simulink model "sg_IK"  (R2021b)
settings: Solver=ode4  StartTime=0.0  StopTime=10  FixedStep=Ts  RelTol=1e-3  EnableMultiTasking=on
model workspace (MAT data in the model file):
  BList = [0  0  0  0  0; 0  1  -1  1  0; -1  0  0  0  1; 0  1.41  -0.25  0  0; -2.61918  0  0  0  0; 0  -2.26918  2.26918  0  0]
  M = [1  0  0  2.61918; 0  1  0  0; 0  0  1  2.24; 0  0  0  1]
  Manual_State_Switch = 0
  Operation_Mode = 2
  SList = [0  0  0  0  0; 0  1  -1  1  0; -1  0  0  0  1; 0  -0.83  1.99  -2.24  0; 0  0  0  0  -2.61918; 0  0.35  -0.35  2.61918  0]
  State_Mode_Selector = 2
  Traj_method = 1
  Winch_EnableHeaveComp = 0
  Winch_NewCmd = 0
  Winch_PosRef = 10
  controlMode = 2
  new_command_traj = 0
  v_max = 0
  x_coordinate_traj = 0
  y_coordinate_traj = 0
  z_coordinate_traj = 0
values from neighbouring files (symbols this model uses):
  Ts = 1e-3    (= 0.001)    [sg_IK_build.m]    (also in sg_IK_startup.m)
libraries: slpidlib x5, slrealtimeutilitieslib x3, slrealtimeiplib x3, dspfdesign x1, simulink x1
(part 1 of 2)
settings Model: SimulationMode=external  Creator=ronnyl10  LastModifiedBy=Thoma
settings SolverCC: ConcurrentTasks=on  AlgebraicLoopSolver=TrustRegion  PositivePriorityOrder=on  AutoInsertRateTranBlk=on  InsertRTBMode=Never (minimum delay)
settings DataIOCC: ExternalInput=ds  SaveFormat=Array  SaveState=on  InspectSignalLogs=on  SignalLoggingName=logsOut
settings OptimizationCC: BlockReduction=off  BooleanDataType=off  OptimizeBlockIOStorage=off  BufferReuse=off  GlobalBufferReuse=off  ExpressionFolding=off  LocalBlockOutputs=off  InitFltsAndDblsToZero=on  OptimizeDataStoreBuffers=off  BusAssignmentInplaceUpdate=off
settings DebuggingCC: SaveWithParameterizedLinksMsg=none  UnderspecifiedInitializationDetection=Classic  MergeDetectMultiDrivingBlocksExec=none  CheckExecutionContextPreStartOutputMsg=on  SignalResolutionControl=TryResolveAllWithWarning  TasksWithSamePriorityMsg=none  SFUnexpectedBacktrackingDiag=warning  SFNoUnconditionalDefaultTransitionDiag=warning  SFExecutionAtInitializationDiag=none  SFMachineParentedDataDiag=warning  ArithmeticOperatorsInVariantConditions=warning
settings HardwareCC: ProdBitPerLong=64  ProdLongLongMode=on  ProdHWDeviceType=Intel->x86-64 (Linux 64)
settings ModelReferenceCC: PropagateSignalLabelsOutOfModel=off
settings SFSimCC: SimUseLocalCustomCode=off  SimTargetLang=C++
settings RTWCC: Description=Simulink Real-Time  SystemTargetFile=slrealtime.tlc  TemplateMakefile=slrealtime_default_tmf  RTWVerbose=off  RTWUseLocalCustomCode=off  Toolchain=Simulink Real-Time Toolchain  BuildConfiguration=Faster Runs  CodeExecutionProfiling=on  TargetLang=C++
settings CodeAppCC: StateflowObjectComments=on
settings SimulinkRealTimeTargetCC: MATLABClassNameForMDSCustomization=Simulink.SoftwareTarget.GRTCustomization  UseGCCFastMath=on
settings ConfigComp: CovEnable=on  RecordCoverage=on  CovMetricSettings=dw  CovSaveCumulativeToWorkspaceVar=on  CovSaveSingleToWorkspaceVar=on  CovModelRefEnable=on  CovExternalEMLEnable=off  CovSFcnEnable=off  PLC_TargetIDE=codesys23  PLC_MultiTBSigbuilderTimeRange=off  PLC_InlineEnumCastFunction=off
settings SimscapeCC: SimscapeLogType=local

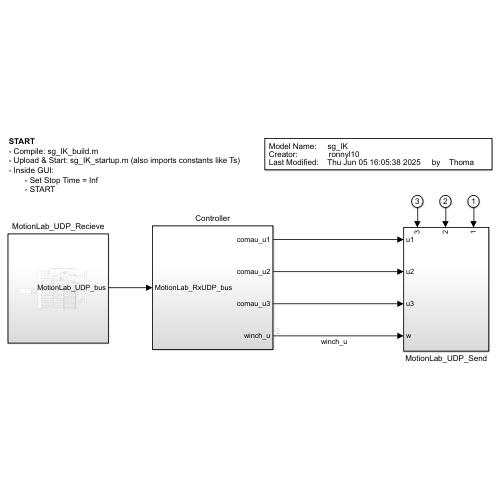
[thumbnail: Simulink's stored preview of the top-level diagram]
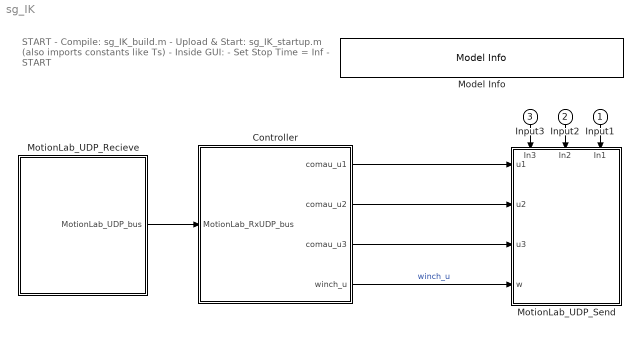
== system sg_IK ==
  note: START
      | - Compile: sg_IK_build.m
      | - Upload & Start: sg_IK_startup.m (also imports constants like Ts)
      | - Inside GUI:
      | - Set Stop Time = Inf
      | - START
  Input1 : Inport  OutDataTypeStr=uint32
  Input2 : Inport  Port=2  OutDataTypeStr=single
  Input3 : Inport  Port=3  OutDataTypeStr=single
  Controller : Subsystem
  Model Info : simulink/Model-Wide Utilities/Model Info  Frame=on  DisplayStringWithTags=|  HorizontalTextAlignment=Left  LeftAlignmentValue=0.02
      | Model Name:     %<ModelName>
      | Creator:              %<Creator>
      | Last Modified:    %<LastModificationDate>     by    %<LastModifiedBy>
  MotionLab_UDP_Recieve : Subsystem
      settings: PortSchema="{\"entries\":[{\"content\":{\"sides\":[{\"content\":{\"connectorIds\":[\"Out1\"]},\"type\":\"ConnectorPlacement.EquallySpacedRectSide\",\"uuid\":\"c59011e9-d1b7-40a2-9e4f-4209006e1514\"},{\"content\":{\"connectorIds\":[],\"side\":\"RIGHT\"},\"type\":\"ConnectorPlacement.EquallySpacedRectSide\",\"uuid\":\"30246177-6108-4738-a92b-25ec176522a5\"},{\"content\":{\"connectorIds\":[],\"side\":\"TOP\"},\"type\":\"ConnectorPlacement.EquallySpacedRectSide\",\"uuid\":\"73bbeb10-9b84-43ee-922e-4b95a3463826\"}]},\"type\":\"ConnectorPlacement.EquallySpacedConnector\",\"uuid\":\"322088d5-facc-406b-b4f7-14c8360d1d37\"}],\"packageUris\":[\"http://schema.mathworks.com/mf0/Connector/R2020b\"],\"version\":\"1.0\"}"
  MotionLab_UDP_Send : Subsystem
      settings: PortSchema="{\"entries\":[{\"content\":{\"sides\":[{\"content\":{\"connectorIds\":[\"In1\",\"In2\",\"In3\"]},\"type\":\"ConnectorPlacement.EquallySpacedRectSide\",\"uuid\":\"2ce4a3a0-ffcc-43d7-9a0a-8eda699e79f7\"},{\"content\":{\"connectorIds\":[],\"side\":\"RIGHT\"},\"type\":\"ConnectorPlacement.EquallySpacedRectSide\",\"uuid\":\"6b0835cb-1c02-4104-b44f-3bd25ad1f1a4\"},{\"content\":{\"connectorIds\":[],\"side\":\"TOP\"},\"type\":\"ConnectorPlacement.EquallySpacedRectSide\",\"uuid\":\"5708f016-a603-4602-bfb0-c60eac1ca3fe\"},{\"content\":{\"connectorIds\":[\"In4\",\"In5\",\"In6\",\"In7\"],\"side\":\"BOTTOM\"},\"type\":\"ConnectorPlacement.EquallySpacedRectSide\",\"uuid\":\"ec76ed57-869b-40d0-9db7-9ec796597bae\"}]},\"type\":\"ConnectorPlacement.EquallySpacedConnector\",\"uuid\":\"dfe3046e-e9d4-4a64-bd13-28ebfaf09d3c\"}],\"packageUris\":[\"http://schema.mathworks.com/mf0/Connector/R2020b\"],\"version\":\"1.0\"}"
  wires:
  Input1/1 -> MotionLab_UDP_Send/1(In1)
  Input3/1 -> MotionLab_UDP_Send/3(In3)
  Input2/1 -> MotionLab_UDP_Send/2(In2)
  Controller/3(comau_u3) -> MotionLab_UDP_Send/6(u3)
  Controller/2(comau_u2) -> MotionLab_UDP_Send/5(u2)
  Controller/1(comau_u1) -> MotionLab_UDP_Send/4(u1)
  Controller/4(winch_u) -> MotionLab_UDP_Send/7(w)  "winch_u"
  MotionLab_UDP_Recieve/1(MotionLab_UDP_bus) -> Controller/1(MotionLab_RxUDP_bus)

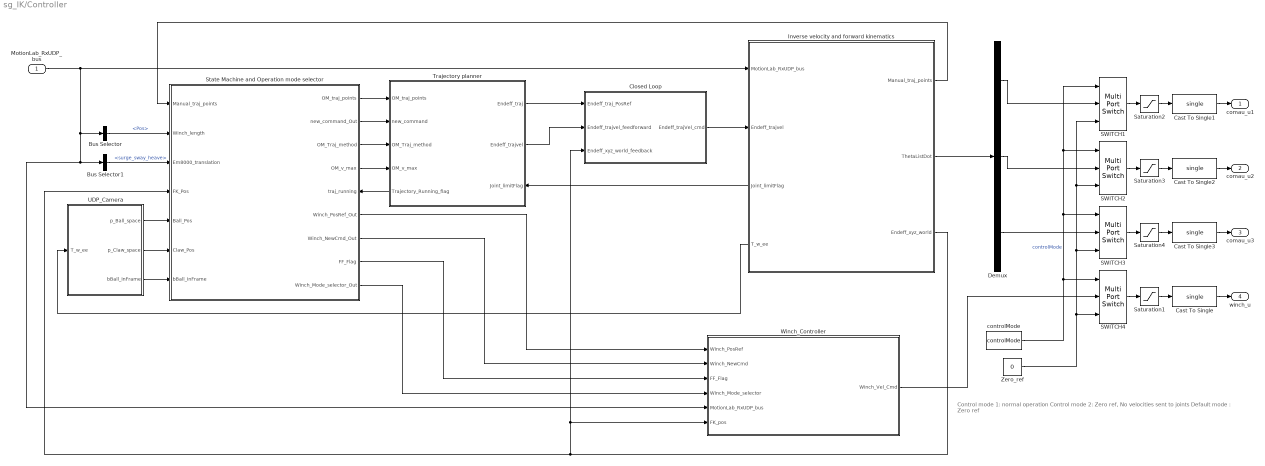
== system sg_IK/Controller ==
  note: Control mode 1: normal operation
      | Control mode 2: Zero ref, No velocities sent to joints
      | Default mode : Zero ref
  MotionLab_RxUDP_bus : Inport
  Bus Selector : BusSelector  OutputSignals=Comau_winch.Pos
  Bus Selector1 : BusSelector  OutputSignals=Em8000.surge_sway_heave
  Cast To Single{,1..3} (4 alike) : DataTypeConversion  OutDataTypeStr=single
  Closed Loop : Subsystem
  Demux : Demux  Outputs=3
  Inverse velocity and forward kinematics : Subsystem
      settings: PortSchema="{\"entries\":[{\"content\":{\"sides\":[{\"content\":{\"connectorIds\":[\"In1\",\"In2\",\"Out4\",\"Out5\"]},\"type\":\"ConnectorPlacement.EquallySpacedRectSide\",\"uuid\":\"551e022a-d0a0-4fc0-a0b4-a546033360d6\"},{\"content\":{\"connectorIds\":[\"Out1\",\"Out2\",\"Out3\"],\"side\":\"RIGHT\"},\"type\":\"ConnectorPlacement.EquallySpacedRectSide\",\"uuid\":\"f9bd0db6-08fd-404e-abaa-5ee6a95abaa6\"},{\"content\":{\"connectorIds\":[],\"side\":\"TOP\"},\"type\":\"ConnectorPlacement.EquallySpacedRectSide\",\"uuid\":\"fe065caa-714c-4067-9577-83ed1adbb3af\"}]},\"type\":\"ConnectorPlacement.EquallySpacedConnector\",\"uuid\":\"f9e419c5-0059-4eec-ae0b-901e5e66b203\"}],\"packageUris\":[\"http://schema.mathworks.com/mf0/Connector/R2020b\"],\"version\":\"1.0\"}"
  SWITCH1 : MultiPortSwitch  Inputs=2
  SWITCH2 : MultiPortSwitch  Inputs=2
  SWITCH3 : MultiPortSwitch  Inputs=2
  SWITCH4 : MultiPortSwitch  Inputs=2  DataPortIndices={1,3}
  Saturation{1..4} (4 alike) : Saturate  UpperLimit=1  LowerLimit=-1
  State Machine and Operation mode selector : Subsystem
      settings: PortSchema="{\"entries\":[{\"content\":{\"sides\":[{\"content\":{\"connectorIds\":[\"In1\",\"In2\",\"In3\",\"In4\",\"In5\",\"In6\",\"In7\"]},\"type\":\"ConnectorPlacement.EquallySpacedRectSide\",\"uuid\":\"2c888d26-e36d-4bcc-8a24-3953247e7d64\"},{\"content\":{\"connectorIds\":[\"Out1\",\"Out2\",\"Out3\",\"Out4\",\"In8\",\"Out5\",\"Out6\",\"Out7\",\"Out8\"],\"side\":\"RIGHT\"},\"type\":\"ConnectorPlacement.EquallySpacedRectSide\",\"uuid\":\"56a7b940-10db-4de5-8f34-3a22dd933015\"},{\"content\":{\"connectorIds\":[],\"side\":\"TOP\"},\"type\":\"ConnectorPlacement.EquallySpacedRectSide\",\"uuid\":\"a958dc8e-1891-4e1e-9098-eeadf2f07291\"}]},\"type\":\"ConnectorPlacement.EquallySpacedConnector\",\"uuid\":\"dcd22044-37ce-4261-aa6a-e53076204f46\"}],\"packageUris\":[\"http://schema.mathworks.com/mf0/Connector/R2020b\"],\"version\":\"1.0\"}"
  Trajectory planner : Subsystem
      settings: PortSchema="{\"entries\":[{\"content\":{\"sides\":[{\"content\":{\"connectorIds\":[\"In1\",\"In2\",\"In3\",\"In4\",\"Out3\"]},\"type\":\"ConnectorPlacement.EquallySpacedRectSide\",\"uuid\":\"e3993239-e7e3-4a56-997d-74b7ac6f065a\"},{\"content\":{\"connectorIds\":[\"Out1\",\"Out2\",\"In5\"],\"side\":\"RIGHT\"},\"type\":\"ConnectorPlacement.EquallySpacedRectSide\",\"uuid\":\"19f001ca-a0d0-47d2-9d98-171e423b1018\"},{\"content\":{\"connectorIds\":[],\"side\":\"TOP\"},\"type\":\"ConnectorPlacement.EquallySpacedRectSide\",\"uuid\":\"ee801cb8-1bce-4750-91c9-73da0ed4f570\"}]},\"type\":\"ConnectorPlacement.EquallySpacedConnector\",\"uuid\":\"affe814f-e012-4d2a-a83d-4eb69c1cbd99\"}],\"packageUris\":[\"http://schema.mathworks.com/mf0/Connector/R2020b\"],\"version\":\"1.0\"}"
  UDP_Camera : Subsystem
  Winch_Controller : Subsystem
  Zero_ref : Constant  Value=0  OutDataTypeStr=double
  controlMode : Constant  Value=controlMode  OutDataTypeStr=double
  comau_u1 : Outport
  comau_u2 : Outport  Port=2
  comau_u3 : Outport  Port=3
  winch_u : Outport  Port=4
  wires:
  Saturation1/1 -> Cast To Single/1
  Zero_ref/1 -> SWITCH1/3, SWITCH2/3, SWITCH3/3, SWITCH4/3
  SWITCH4/1 -> Saturation1/1
  SWITCH1/1 -> Saturation2/1
  SWITCH2/1 -> Saturation3/1
  SWITCH3/1 -> Saturation4/1
  controlMode/1 -> SWITCH1/1, SWITCH2/1, SWITCH3/1, SWITCH4/1  "controlMode"
  Cast To Single/1 -> winch_u/1
  Cast To Single3/1 -> comau_u3/1
  Saturation4/1 -> Cast To Single3/1
  Saturation3/1 -> Cast To Single2/1
  Cast To Single2/1 -> comau_u2/1
  Saturation2/1 -> Cast To Single1/1
  Cast To Single1/1 -> comau_u1/1
  Demux/1 -> SWITCH1/2
  Demux/2 -> SWITCH2/2
  Demux/3 -> SWITCH3/2
  Winch_Controller/1(Winch_Vel_Cmd) -> SWITCH4/2
  Inverse velocity and forward kinematics/3(Endeff_xyz_world) -> Winch_Controller/6(FK_pos), Closed Loop/3(Endeff_xyz_world_feedback), State Machine and Operation mode selector/4(FK_Pos)
  MotionLab_RxUDP_bus/1 -> Winch_Controller/5(MotionLab_RxUDP_bus), Bus Selector1/1, Bus Selector/1, Inverse velocity and forward kinematics/1(MotionLab_RxUDP_bus)
  Inverse velocity and forward kinematics/2(ThetaListDot) -> Demux/1
  Inverse velocity and forward kinematics/4(Joint_limitFlag) -> Trajectory planner/5(Joint_limitFlag)
  Trajectory planner/2(Endeff_trajvel) -> Closed Loop/2(Endeff_trajvel_feedforward)
  Inverse velocity and forward kinematics/1(Manual_traj_points) -> State Machine and Operation mode selector/1(Manual_traj_points)
  Trajectory planner/3(Trajectory_Running_flag) -> State Machine and Operation mode selector/8(traj_running)
  UDP_Camera/1(p_Ball_space) -> State Machine and Operation mode selector/5(Ball_Pos)
  UDP_Camera/2(p_Claw_space) -> State Machine and Operation mode selector/6(Claw_Pos)
  UDP_Camera/3(bBall_InFrame) -> State Machine and Operation mode selector/7(bBall_InFrame)
  State Machine and Operation mode selector/1(OM_traj_points) -> Trajectory planner/1(OM_traj_points)
  State Machine and Operation mode selector/2(new_command_Out) -> Trajectory planner/2(new_command)
  State Machine and Operation mode selector/3(OM_Traj_method) -> Trajectory planner/3(OM_Traj_method)
  State Machine and Operation mode selector/4(OM_v_max) -> Trajectory planner/4(OM_v_max)
  State Machine and Operation mode selector/5(Winch_PosRef_Out) -> Winch_Controller/1(Winch_PosRef)
  State Machine and Operation mode selector/6(Winch_NewCmd_Out) -> Winch_Controller/2(Winch_NewCmd)
  State Machine and Operation mode selector/7(FF_Flag) -> Winch_Controller/3(FF_Flag)
  Bus Selector/1 -> State Machine and Operation mode selector/2(Winch_length)  "<Pos>"
  Inverse velocity and forward kinematics/5(T_w_ee) -> UDP_Camera/1(T_w_ee)
  State Machine and Operation mode selector/8(Winch_Mode_selector_Out) -> Winch_Controller/4(Winch_Mode_selector)
  Bus Selector1/1 -> State Machine and Operation mode selector/3(Em8000_translation)  "<surge_sway_heave>"
  Closed Loop/1(Endeff_trajVel_cmd) -> Inverse velocity and forward kinematics/2(Endeff_trajvel)
  Trajectory planner/1(Endeff_traj) -> Closed Loop/1(Endeff_traj_PosRef)

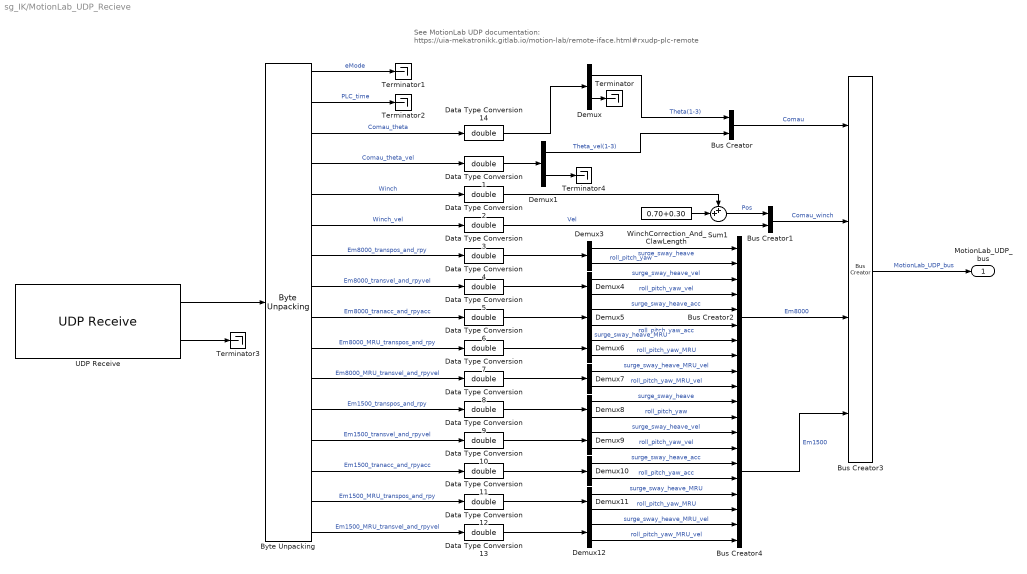
== system sg_IK/MotionLab_UDP_Recieve ==
  note: See MotionLab UDP documentation:
      | https://uia-mekatronikk.gitlab.io/motion-lab/remote-iface.html#rxudp-plc-remote
  Bus Creator : BusCreator  Inputs=2
  Bus Creator1 : BusCreator  Inputs=2
  Bus Creator2 : BusCreator  Inputs=10
  Bus Creator3 : BusCreator  Inputs=4
  Bus Creator4 : BusCreator  Inputs=10
  Byte Unpacking : slrealtimeutilitieslib/Byte Unpacking  MaskUnpackedDataTypes={'uint32', 'single', 'single', 'single', 'single', 'single', 'single', 'single', 'single', 'single', 'single', 'single', 'single', 'single', 'single', 'single'}  MaskUnpackedDataSizes={[1], [1], [6], [6], [1], [1], [6], [6], [6], [6], [6], [6], [6], [6], [6], [6]}  MaskAlignment=1
      settings: SourceProductBaseCode=XP
  Data Type Conversion{1..14} (14 alike) : DataTypeConversion  OutDataTypeStr=double
  Demux{,1,3..12} (12 alike) : Demux  Outputs=2
  Sum1 : Sum  Inputs=++|
  Terminator{,1..4} (5 alike) : Terminator
  UDP Receive : slrealtimeiplib/UDP Receive  useHostTargetConn=on  ipAddress=192.168.90.60  localPort=50060  rcvWidth=304  rcvFmAny=on  fmAddress=192.168.90.50  sampleTime=Ts
      settings: SourceProductBaseCode=XP
  WinchCorrection_And_ClawLength : Constant  Value=0.70+0.30
  MotionLab_UDP_bus : Outport
  wires:
  Byte Unpacking/14 -> Data Type Conversion11/1  "Em1500_tranacc_and_rpyacc"
  Byte Unpacking/11 -> Data Type Conversion8/1  "Em8000_MRU_transvel_and_rpyvel"
  Byte Unpacking/12 -> Data Type Conversion9/1  "Em1500_transpos_and_rpy"
  Byte Unpacking/8 -> Data Type Conversion5/1  "Em8000_transvel_and_rpyvel"
  Demux5/1 -> Bus Creator2/5  "surge_sway_heave_acc"
  Byte Unpacking/2 -> Terminator2/1  "PLC_time"
  Data Type Conversion6/1 -> Demux5/1
  Byte Unpacking/16 -> Data Type Conversion13/1  "Em1500_MRU_transvel_and_rpyvel"
  Byte Unpacking/3 -> Data Type Conversion14/1  "Comau_theta"
  Demux9/1 -> Bus Creator4/3  "surge_sway_heave_vel"
  Data Type Conversion7/1 -> Demux6/1
  Byte Unpacking/4 -> Data Type Conversion1/1  "Comau_theta_vel"
  Data Type Conversion12/1 -> Demux11/1
  Data Type Conversion13/1 -> Demux12/1
  Byte Unpacking/5 -> Data Type Conversion2/1  "Winch"
  Data Type Conversion11/1 -> Demux10/1
  Demux4/1 -> Bus Creator2/3  "surge_sway_heave_vel"
  Byte Unpacking/13 -> Data Type Conversion10/1  "Em1500_transvel_and_rpyvel"
  Byte Unpacking/9 -> Data Type Conversion6/1  "Em8000_tranacc_and_rpyacc"
  Data Type Conversion8/1 -> Demux7/1
  Data Type Conversion5/1 -> Demux4/1
  Demux12/2 -> Bus Creator4/10  "roll_pitch_yaw_MRU_vel"
  Data Type Conversion9/1 -> Demux8/1
  Byte Unpacking/7 -> Data Type Conversion4/1  "Em8000_transpos_and_rpy"
  Bus Creator3/1 -> MotionLab_UDP_bus/1  "MotionLab_UDP_bus"
  Data Type Conversion3/1 -> Bus Creator1/2  "Vel"
  Byte Unpacking/1 -> Terminator1/1  "eMode"
  Demux9/2 -> Bus Creator4/4  "roll_pitch_yaw_vel"
  Demux7/2 -> Bus Creator2/10  "roll_pitch_yaw_MRU_vel"
  Demux8/2 -> Bus Creator4/2  "roll_pitch_yaw"
  Data Type Conversion4/1 -> Demux3/1
  UDP Receive/2 -> Terminator3/1
  Byte Unpacking/10 -> Data Type Conversion7/1  "Em8000_MRU_transpos_and_rpy"
  Bus Creator1/1 -> Bus Creator3/2  "Comau_winch"
  Demux6/2 -> Bus Creator2/8  "roll_pitch_yaw_MRU"
  Demux12/1 -> Bus Creator4/9  "surge_sway_heave_MRU_vel"
  Demux5/2 -> Bus Creator2/6  "roll_pitch_yaw_acc"
  Demux11/2 -> Bus Creator4/8  "roll_pitch_yaw_MRU"
  Byte Unpacking/6 -> Data Type Conversion3/1  "Winch_vel"
  Demux11/1 -> Bus Creator4/7  "surge_sway_heave_MRU"
  Demux10/1 -> Bus Creator4/5  "surge_sway_heave_acc"
  Demux3/1 -> Bus Creator2/1  "surge_sway_heave"
  Demux10/2 -> Bus Creator4/6  "roll_pitch_yaw_acc"
  Demux7/1 -> Bus Creator2/9  "surge_sway_heave_MRU_vel"
  Bus Creator2/1 -> Bus Creator3/3  "Em8000"
  Demux/2 -> Terminator/1
  Sum1/1 -> Bus Creator1/1  "Pos"
  Bus Creator4/1 -> Bus Creator3/4  "Em1500"
  Data Type Conversion10/1 -> Demux9/1
  WinchCorrection_And_ClawLength/1 -> Sum1/2
  Demux4/2 -> Bus Creator2/4  "roll_pitch_yaw_vel"
  Byte Unpacking/15 -> Data Type Conversion12/1  "Em1500_MRU_transpos_and_rpy"
  Demux3/2 -> Bus Creator2/2  "roll_pitch_yaw"
  Demux1/1 -> Bus Creator/2  "Theta_vel(1-3)"
  UDP Receive/1 -> Byte Unpacking/1
  Bus Creator/1 -> Bus Creator3/1  "Comau"
  Demux/1 -> Bus Creator/1  "Theta(1-3)"
  Demux8/1 -> Bus Creator4/1  "surge_sway_heave"
  Data Type Conversion14/1 -> Demux/1
  Demux6/1 -> Bus Creator2/7  "surge_sway_heave_MRU"
  Data Type Conversion2/1 -> Sum1/1
  Demux1/2 -> Terminator4/1
  Data Type Conversion1/1 -> Demux1/1

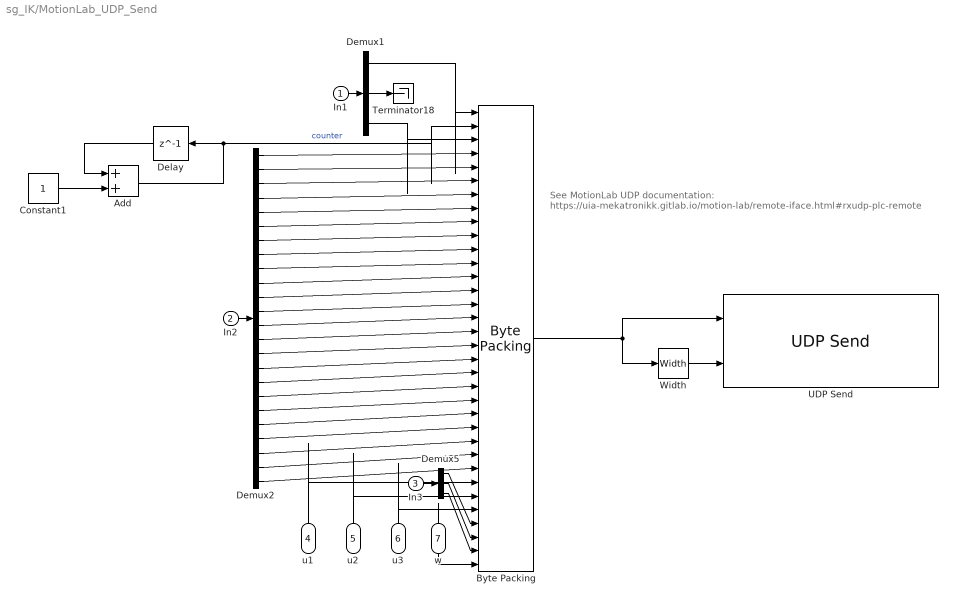
== system sg_IK/MotionLab_UDP_Send ==
  note: See MotionLab UDP documentation:
      | https://uia-mekatronikk.gitlab.io/motion-lab/remote-iface.html#rxudp-plc-remote
  In1 : Inport
  In2 : Inport  Port=2
  In3 : Inport  Port=3
  u1 : Inport  Port=4
  u2 : Inport  Port=5
  u3 : Inport  Port=6
  w : Inport  Port=7
  Add : Sum
  Byte Packing : slrealtimeutilitieslib/Byte Packing  MaskPackedDataType=uint8  MaskUnpackedDataTypes={'uint32', 'uint32', 'uint32', 'single', 'single', 'single', 'single', 'single', 'single', 'single', 'single', 'single', 'single', 'single', 'single', 'single', 'single', 'single', 'single', 'single', 'single', 'single', 'single', 'single', 'single', 'single', 'single', 'single', 'single', 'single', 'single', 'single', 'single', 'single'}  MaskAlignment=1
  Constant1 : Constant  OutDataTypeStr=uint32
  Delay : Delay  DelayLength=1
  Demux1 : Demux  Outputs=3
  Demux2 : Demux  Outputs=24
  Demux5 : Demux  Outputs=3
  Terminator18 : Terminator
  UDP Send : slrealtimeiplib/UDP Send  useHostTargetConn=on  toAddress=192.168.90.50  toPort=50050  sampleTime=Ts  localPort=11000
      settings: SourceProductBaseCode=XP
  Width : Width
  wires:
  Demux2/19 -> Byte Packing/22
  Demux2/21 -> Byte Packing/24
  u3/1 -> Byte Packing/30
  Demux2/2 -> Byte Packing/5
  u2/1 -> Byte Packing/29
  Demux5/1 -> Byte Packing/31
  Demux5/2 -> Byte Packing/32
  Demux1/3 -> Byte Packing/3
  In2/1 -> Demux2/1
  Demux2/22 -> Byte Packing/25
  Demux2/1 -> Byte Packing/4
  Demux2/15 -> Byte Packing/18
  Demux2/18 -> Byte Packing/21
  Delay/1 -> Add/1
  Demux2/24 -> Byte Packing/27
  Demux1/2 -> Terminator18/1
  In1/1 -> Demux1/1
  Demux2/5 -> Byte Packing/8
  Add/1 -> Byte Packing/2, Delay/1  "counter"
  Constant1/1 -> Add/2
  Demux2/6 -> Byte Packing/9
  Demux2/9 -> Byte Packing/12
  Demux2/10 -> Byte Packing/13
  Demux2/20 -> Byte Packing/23
  Demux2/8 -> Byte Packing/11
  Demux2/12 -> Byte Packing/15
  Demux2/23 -> Byte Packing/26
  Demux2/16 -> Byte Packing/19
  Demux1/1 -> Byte Packing/1
  Demux5/3 -> Byte Packing/33
  Demux2/3 -> Byte Packing/6
  Demux2/11 -> Byte Packing/14
  Demux2/7 -> Byte Packing/10
  Demux2/4 -> Byte Packing/7
  Demux2/13 -> Byte Packing/16
  Demux2/17 -> Byte Packing/20
  Demux2/14 -> Byte Packing/17
  u1/1 -> Byte Packing/28
  In3/1 -> Demux5/1
  w/1 -> Byte Packing/34
  Byte Packing/1 -> Width/1, UDP Send/1
  Width/1 -> UDP Send/2

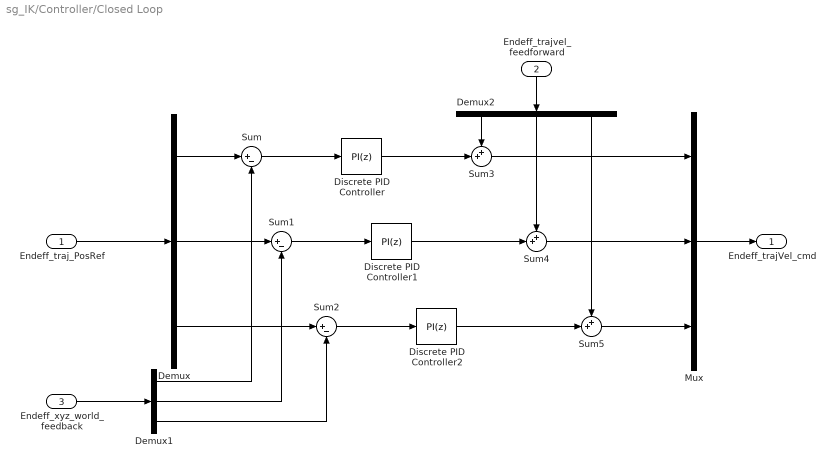
== system sg_IK/Controller/Closed Loop ==
  Endeff_traj_PosRef : Inport
  Endeff_trajvel_feedforward : Inport  Port=2
  Endeff_xyz_world_feedback : Inport  Port=3
  Demux : Demux  Outputs=3
  Demux1 : Demux  Outputs=3
  Demux2 : Demux  Outputs=3
  Discrete PID Controller : slpidlib/PID Controller  Controller=PI  Form=Parallel  TimeDomain=Discrete-time  UseExternalTs=off  SampleTime=Ts  IntegratorMethod=Forward Euler  FilterMethod=Forward Euler  ControllerParametersSource=internal  P=0.25  I=0.0125  D=0  UseFilter=on  N=100  TunerSelectOption=Transfer Function Based (PID Tuner App)  InitialConditionSource=internal  InitialConditionForIntegrator=0  InitialConditionForFilter=0  DifferentiatorICPrevScaledInput=0  ExternalReset=none  TrackingMode=off  Kt=1  LimitOutput=on  SatLimitsSource=internal  UpperSaturationLimit=0.2  LowerSaturationLimit=-0.2  LinearizeAsGain=off  AntiWindupMode=none  Kb=1  POutMin=[]  POutMax=[]  IOutMin=[]  IOutMax=[]  DOutMin=[]  DOutMax=[]  NOutMin=[]  NOutMax=[]  SumOutMin=[]  SumOutMax=[]  SaturationOutMin=[]  SaturationOutMax=[]  PParamMin=[]  PParamMax=[]  IParamMin=[]  IParamMax=[]  DParamMin=[]  DParamMax=[]  NParamMin=[]  NParamMax=[]  KbParamMin=[]  KbParamMax=[]  KtParamMin=[]  KtParamMax=[]  KbOutMin=[]  KbOutMax=[]  KtOutMin=[]  KtOutMax=[]  IntegratorOutMin=[]  IntegratorOutMax=[]  FilterOutMin=[]  FilterOutMax=[]  SumI1OutMin=[]  SumI1OutMax=[]  SumI2OutMin=[]  SumI2OutMax=[]  SumI3OutMin=[]  SumI3OutMax=[]  SumI4OutMin=[]  SumI4OutMax=[]  SumDOutMin=[]  SumDOutMax=[]  DifferentiatorOutMin=[]  DifferentiatorOutMax=[]  FilterDiffOutCoefMin=[]  FilterDiffOutCoefMax=[]  ReciprocalOutMin=[]  ReciprocalOutMax=[]  SumDenOutMin=[]  SumDenOutMax=[]  SumNumOutMin=[]  SumNumOutMax=[]  DivideOutMin=[]  DivideOutMax=[]  UdiffTsProdOutMin=[]  UdiffTsProdOutMax=[]  NTsProdOutMin=[]  NTsProdOutMax=[]  UintegralTsProdOutMin=[]  UintegralTsProdOutMax=[]  UngainTsProdOutMin=[]  UngainTsProdOutMax=[]  FilterDenConstantOutDataTypeStr=Inherit: Inherit via back propagation  FilterDenConstantOutMin=[]  FilterDenConstantOutMax=[]  PCopyOutDataTypeStr=Inherit: Inherit via back propagation  PCopyOutMin=[]  PCopyOutMax=[]  NCopyOutDataTypeStr=Inherit: Inherit via back propagation  NCopyOutMin=[]  NCopyOutMax=[]  IntegratorContinuousStateAttributes=''  IntegratorStateMustResolveToSignalObject=off  IntegratorRTWStateStorageClass=Auto  FilterContinuousStateAttributes=''  FilterStateMustResolveToSignalObject=off  FilterRTWStateStorageClass=Auto  ParallelPVariant=InternalParameters  IdealPVariant=Disabled  IVariant=InternalParameters  DVariant=Disabled  IntegratorVariant=Discrete  SatVariant=Enabled  AWVariant=Passthrough  PCopyVariant=Disabled  TRVariant=Disabled  FdbkBlocksVariant=Forward  IdealPFdbkVariant=Disabled  SatFdbkVariant=Disabled  DerivativeFilterVariant=Disabled  NVariant=Disabled  NCopyVariant=Disabled_SignalSpec  FilterICVariant=Disabled  IntegratorICVariant=InternalICs  ExternalResetVariant=Disabled  TRSumVariant=Passthrough  SumFdbkVariant=Disabled  SumVariant=Sum_PI  TsampFilterVariant=InternalTs  TsampNgainVariant=Passthrough  TsampIntegralVariant=Passthrough  ExternalSaturationOutDataTypeStr=Inherit: Same as second input
  Discrete PID Controller1 : slpidlib/PID Controller  Controller=PI  Form=Parallel  TimeDomain=Discrete-time  UseExternalTs=off  SampleTime=Ts  IntegratorMethod=Forward Euler  FilterMethod=Forward Euler  ControllerParametersSource=internal  P=0.25  I=0.0125  D=0  UseFilter=on  N=100  TunerSelectOption=Transfer Function Based (PID Tuner App)  InitialConditionSource=internal  InitialConditionForIntegrator=0  InitialConditionForFilter=0  DifferentiatorICPrevScaledInput=0  ExternalReset=none  TrackingMode=off  Kt=1  LimitOutput=on  SatLimitsSource=internal  UpperSaturationLimit=0.2  LowerSaturationLimit=-0.2  LinearizeAsGain=off  AntiWindupMode=none  Kb=1  POutMin=[]  POutMax=[]  IOutMin=[]  IOutMax=[]  DOutMin=[]  DOutMax=[]  NOutMin=[]  NOutMax=[]  SumOutMin=[]  SumOutMax=[]  SaturationOutMin=[]  SaturationOutMax=[]  PParamMin=[]  PParamMax=[]  IParamMin=[]  IParamMax=[]  DParamMin=[]  DParamMax=[]  NParamMin=[]  NParamMax=[]  KbParamMin=[]  KbParamMax=[]  KtParamMin=[]  KtParamMax=[]  KbOutMin=[]  KbOutMax=[]  KtOutMin=[]  KtOutMax=[]  IntegratorOutMin=[]  IntegratorOutMax=[]  FilterOutMin=[]  FilterOutMax=[]  SumI1OutMin=[]  SumI1OutMax=[]  SumI2OutMin=[]  SumI2OutMax=[]  SumI3OutMin=[]  SumI3OutMax=[]  SumI4OutMin=[]  SumI4OutMax=[]  SumDOutMin=[]  SumDOutMax=[]  DifferentiatorOutMin=[]  DifferentiatorOutMax=[]  FilterDiffOutCoefMin=[]  FilterDiffOutCoefMax=[]  ReciprocalOutMin=[]  ReciprocalOutMax=[]  SumDenOutMin=[]  SumDenOutMax=[]  SumNumOutMin=[]  SumNumOutMax=[]  DivideOutMin=[]  DivideOutMax=[]  UdiffTsProdOutMin=[]  UdiffTsProdOutMax=[]  NTsProdOutMin=[]  NTsProdOutMax=[]  UintegralTsProdOutMin=[]  UintegralTsProdOutMax=[]  UngainTsProdOutMin=[]  UngainTsProdOutMax=[]  FilterDenConstantOutDataTypeStr=Inherit: Inherit via back propagation  FilterDenConstantOutMin=[]  FilterDenConstantOutMax=[]  PCopyOutDataTypeStr=Inherit: Inherit via back propagation  PCopyOutMin=[]  PCopyOutMax=[]  NCopyOutDataTypeStr=Inherit: Inherit via back propagation  NCopyOutMin=[]  NCopyOutMax=[]  IntegratorContinuousStateAttributes=''  IntegratorStateMustResolveToSignalObject=off  IntegratorRTWStateStorageClass=Auto  FilterContinuousStateAttributes=''  FilterStateMustResolveToSignalObject=off  FilterRTWStateStorageClass=Auto  ParallelPVariant=InternalParameters  IdealPVariant=Disabled  IVariant=InternalParameters  DVariant=Disabled  IntegratorVariant=Discrete  SatVariant=Enabled  AWVariant=Passthrough  PCopyVariant=Disabled  TRVariant=Disabled  FdbkBlocksVariant=Forward  IdealPFdbkVariant=Disabled  SatFdbkVariant=Disabled  DerivativeFilterVariant=Disabled  NVariant=Disabled  NCopyVariant=Disabled_SignalSpec  FilterICVariant=Disabled  IntegratorICVariant=InternalICs  ExternalResetVariant=Disabled  TRSumVariant=Passthrough  SumFdbkVariant=Disabled  SumVariant=Sum_PI  TsampFilterVariant=InternalTs  TsampNgainVariant=Passthrough  TsampIntegralVariant=Passthrough  ExternalSaturationOutDataTypeStr=Inherit: Same as second input
  Discrete PID Controller2 : slpidlib/PID Controller  Controller=PI  Form=Parallel  TimeDomain=Discrete-time  UseExternalTs=off  SampleTime=Ts  IntegratorMethod=Forward Euler  FilterMethod=Forward Euler  ControllerParametersSource=internal  P=0.25  I=0.0125  D=0  UseFilter=on  N=100  TunerSelectOption=Transfer Function Based (PID Tuner App)  InitialConditionSource=internal  InitialConditionForIntegrator=0  InitialConditionForFilter=0  DifferentiatorICPrevScaledInput=0  ExternalReset=none  TrackingMode=off  Kt=1  LimitOutput=on  SatLimitsSource=internal  UpperSaturationLimit=0.2  LowerSaturationLimit=-0.2  LinearizeAsGain=off  AntiWindupMode=none  Kb=1  POutMin=[]  POutMax=[]  IOutMin=[]  IOutMax=[]  DOutMin=[]  DOutMax=[]  NOutMin=[]  NOutMax=[]  SumOutMin=[]  SumOutMax=[]  SaturationOutMin=[]  SaturationOutMax=[]  PParamMin=[]  PParamMax=[]  IParamMin=[]  IParamMax=[]  DParamMin=[]  DParamMax=[]  NParamMin=[]  NParamMax=[]  KbParamMin=[]  KbParamMax=[]  KtParamMin=[]  KtParamMax=[]  KbOutMin=[]  KbOutMax=[]  KtOutMin=[]  KtOutMax=[]  IntegratorOutMin=[]  IntegratorOutMax=[]  FilterOutMin=[]  FilterOutMax=[]  SumI1OutMin=[]  SumI1OutMax=[]  SumI2OutMin=[]  SumI2OutMax=[]  SumI3OutMin=[]  SumI3OutMax=[]  SumI4OutMin=[]  SumI4OutMax=[]  SumDOutMin=[]  SumDOutMax=[]  DifferentiatorOutMin=[]  DifferentiatorOutMax=[]  FilterDiffOutCoefMin=[]  FilterDiffOutCoefMax=[]  ReciprocalOutMin=[]  ReciprocalOutMax=[]  SumDenOutMin=[]  SumDenOutMax=[]  SumNumOutMin=[]  SumNumOutMax=[]  DivideOutMin=[]  DivideOutMax=[]  UdiffTsProdOutMin=[]  UdiffTsProdOutMax=[]  NTsProdOutMin=[]  NTsProdOutMax=[]  UintegralTsProdOutMin=[]  UintegralTsProdOutMax=[]  UngainTsProdOutMin=[]  UngainTsProdOutMax=[]  FilterDenConstantOutDataTypeStr=Inherit: Inherit via back propagation  FilterDenConstantOutMin=[]  FilterDenConstantOutMax=[]  PCopyOutDataTypeStr=Inherit: Inherit via back propagation  PCopyOutMin=[]  PCopyOutMax=[]  NCopyOutDataTypeStr=Inherit: Inherit via back propagation  NCopyOutMin=[]  NCopyOutMax=[]  IntegratorContinuousStateAttributes=''  IntegratorStateMustResolveToSignalObject=off  IntegratorRTWStateStorageClass=Auto  FilterContinuousStateAttributes=''  FilterStateMustResolveToSignalObject=off  FilterRTWStateStorageClass=Auto  ParallelPVariant=InternalParameters  IdealPVariant=Disabled  IVariant=InternalParameters  DVariant=Disabled  IntegratorVariant=Discrete  SatVariant=Enabled  AWVariant=Passthrough  PCopyVariant=Disabled  TRVariant=Disabled  FdbkBlocksVariant=Forward  IdealPFdbkVariant=Disabled  SatFdbkVariant=Disabled  DerivativeFilterVariant=Disabled  NVariant=Disabled  NCopyVariant=Disabled_SignalSpec  FilterICVariant=Disabled  IntegratorICVariant=InternalICs  ExternalResetVariant=Disabled  TRSumVariant=Passthrough  SumFdbkVariant=Disabled  SumVariant=Sum_PI  TsampFilterVariant=InternalTs  TsampNgainVariant=Passthrough  TsampIntegralVariant=Passthrough  ExternalSaturationOutDataTypeStr=Inherit: Same as second input
  Mux : Mux  Inputs=3
  Sum : Sum  Inputs=|+-
  Sum1 : Sum  Inputs=|+-
  Sum2 : Sum  Inputs=|+-
  Sum3 : Sum  Inputs=++|
  Sum4 : Sum  Inputs=++|
  Sum5 : Sum  Inputs=++|
  Endeff_trajVel_cmd : Outport
  wires:
  Endeff_traj_PosRef/1 -> Demux/1
  Sum/1 -> Discrete PID Controller/1
  Endeff_xyz_world_feedback/1 -> Demux1/1
  Demux1/1 -> Sum/2
  Sum1/1 -> Discrete PID Controller1/1
  Sum2/1 -> Discrete PID Controller2/1
  Demux1/2 -> Sum1/2
  Demux1/3 -> Sum2/2
  Demux/3 -> Sum2/1
  Demux/2 -> Sum1/1
  Demux/1 -> Sum/1
  Discrete PID Controller/1 -> Sum3/2
  Endeff_trajvel_feedforward/1 -> Demux2/1
  Discrete PID Controller1/1 -> Sum4/2
  Discrete PID Controller2/1 -> Sum5/2
  Mux/1 -> Endeff_trajVel_cmd/1
  Sum4/1 -> Mux/2
  Sum3/1 -> Mux/1
  Sum5/1 -> Mux/3
  Demux2/1 -> Sum3/1
  Demux2/2 -> Sum4/1
  Demux2/3 -> Sum5/1

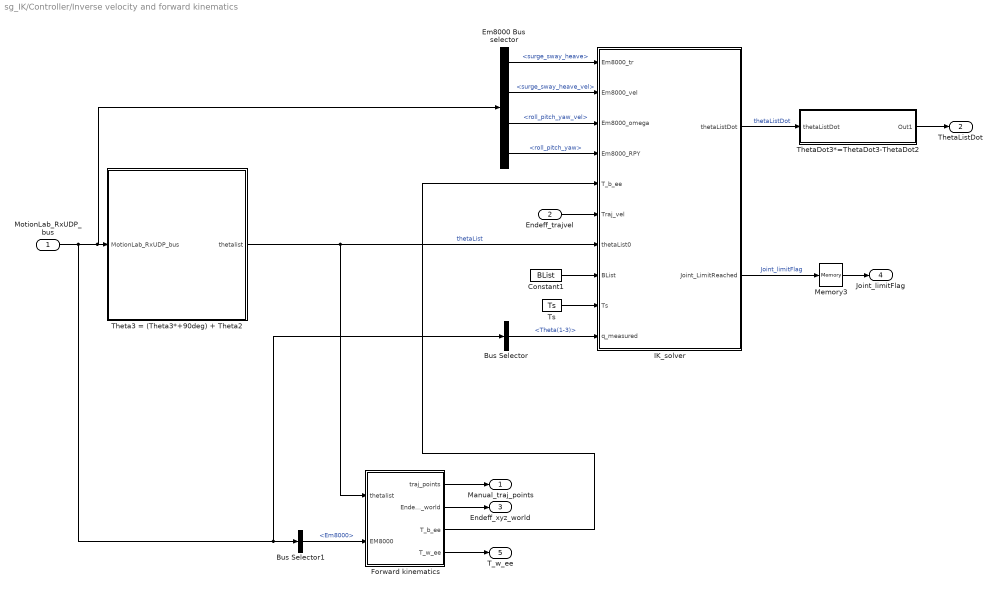
== system sg_IK/Controller/Inverse velocity and forward kinematics ==
  MotionLab_RxUDP_bus : Inport
  Endeff_trajvel : Inport  Port=2
  Bus Selector : BusSelector  OutputSignals=Comau.Theta(1-3)
  Bus Selector1 : BusSelector  OutputSignals=Em8000
  Constant1 : Constant  Value=BList
  Em8000 Bus selector : BusSelector  OutputSignals=Em8000.surge_sway_heave,Em8000.surge_sway_heave_vel,Em8000.roll_pitch_yaw_vel,Em8000.roll_pitch_yaw
  Forward kinematics : Subsystem
  IK_solver : MATLAB Function  TreatAsAtomicUnit=on
  Memory3 : Memory
  Theta3 = (Theta3*+90deg) + Theta2 : Subsystem
  ThetaDot3*=ThetaDot3-ThetaDot2 : Subsystem
  Ts : Constant  Value=Ts
  Manual_traj_points : Outport
  ThetaListDot : Outport  Port=2
  Endeff_xyz_world : Outport  Port=3
  Joint_limitFlag : Outport  Port=4
  T_w_ee : Outport  Port=5
  wires:
  Ts/1 -> IK_solver/9(Ts)
  Theta3 = (Theta3*+90deg) + Theta2/1(thetalist) -> Forward kinematics/1(thetalist), IK_solver/7(thetaList0)  "thetaList"
  Forward kinematics/3(T_b_ee) -> IK_solver/5(T_b_ee)
  IK_solver/1(thetaListDot) -> ThetaDot3*=ThetaDot3-ThetaDot2/1(thetaListDot)  "thetaListDot"
  ThetaDot3*=ThetaDot3-ThetaDot2/1(Out1) -> ThetaListDot/1
  Constant1/1 -> IK_solver/8(BList)
  Em8000 Bus selector/3 -> IK_solver/3(Em8000_omega)  "<roll_pitch_yaw_vel>"
  IK_solver/2(Joint_LimitReached) -> Memory3/1  "Joint_limitFlag"
  Em8000 Bus selector/1 -> IK_solver/1(Em8000_tr)  "<surge_sway_heave>"
  Memory3/1 -> Joint_limitFlag/1
  Em8000 Bus selector/2 -> IK_solver/2(Em8000_vel)  "<surge_sway_heave_vel>"
  MotionLab_RxUDP_bus/1 -> Theta3 = (Theta3*+90deg) + Theta2/1(MotionLab_RxUDP_bus), Em8000 Bus selector/1, Bus Selector/1, Bus Selector1/1
  Bus Selector1/1 -> Forward kinematics/2(EM8000)  "<Em8000>"
  Forward kinematics/2(Endeff_xyz_world) -> Endeff_xyz_world/1
  Em8000 Bus selector/4 -> IK_solver/4(Em8000_RPY)  "<roll_pitch_yaw>"
  Endeff_trajvel/1 -> IK_solver/6(Traj_vel)
  Forward kinematics/1(traj_points) -> Manual_traj_points/1
  Bus Selector/1 -> IK_solver/10(q_measured)  "<Theta(1-3)>"
  Forward kinematics/4(T_w_ee) -> T_w_ee/1

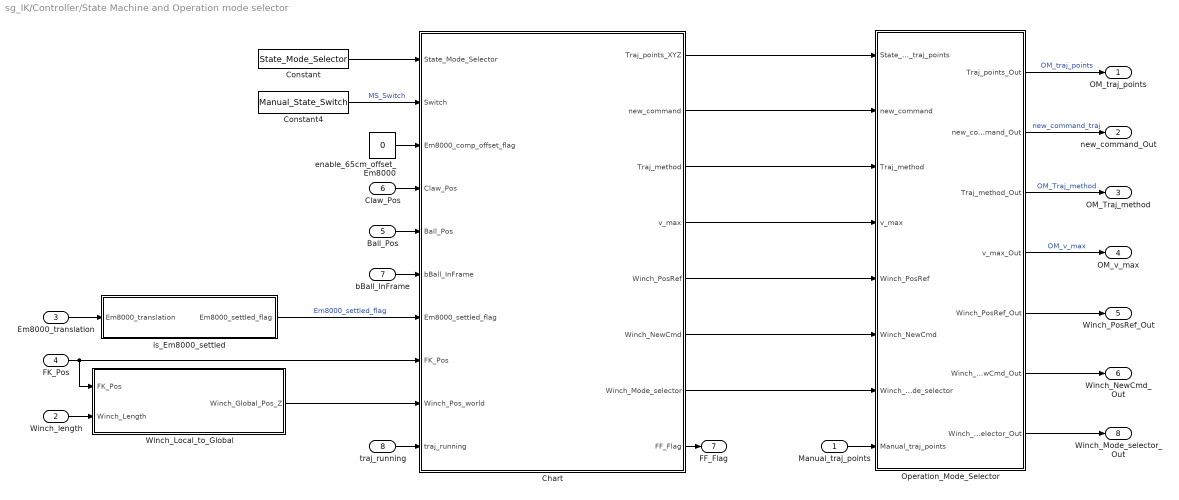
== system sg_IK/Controller/State Machine and Operation mode selector ==
  Manual_traj_points : Inport
  Winch_length : Inport  Port=2
  Em8000_translation : Inport  Port=3
  FK_Pos : Inport  Port=4
  Ball_Pos : Inport  Port=5
  Claw_Pos : Inport  Port=6
  bBall_InFrame : Inport  Port=7
  traj_running : Inport  Port=8
  Chart : Stateflow chart  TreatAsAtomicUnit=on
      settings: PortSchema="{\"entries\":[{\"content\":{\"sides\":[{\"content\":{\"connectorIds\":[\"In1\",\"In2\",\"In3\",\"In5\",\"In8\",\"In6\",\"In7\",\"In4\",\"In9\",\"In10\"]},\"type\":\"ConnectorPlacement.EquallySpacedRectSide\",\"uuid\":\"4efafd74-82d1-44f1-a055-c18d6c912383\"},{\"content\":{\"connectorIds\":[\"Out1\",\"Out2\",\"Out3\",\"Out4\",\"Out6\",\"Out5\",\"Out7\",\"Out8\"],\"side\":\"RIGHT\"},\"type\":\"ConnectorPlacement.EquallySpacedRectSide\",\"uuid\":\"5371acfb-0eb7-4cc0-8895-01a809823e9a\"},{\"content\":{\"connectorIds\":[],\"side\":\"TOP\"},\"type\":\"ConnectorPlacement.EquallySpacedRectSide\",\"uuid\":\"d70aff37-3d55-422d-a0a5-3282bb577d57\"}]},\"type\":\"ConnectorPlacement.EquallySpacedConnector\",\"uuid\":\"f8da4380-4301-4a58-af79-e06d3d1a2e95\"}],\"packageUris\":[\"http://schema.mathworks.com/mf0/Connector/R2020b\"],\"version\":\"1.0\"}"
  Constant : Constant  Value=State_Mode_Selector
  Constant4 : Constant  Value=Manual_State_Switch
  Operation_Mode_Selector : Subsystem
  Winch_Local_to_Global : MATLAB Function  TreatAsAtomicUnit=on
  enable_65cm_offset_Em8000 : Constant  Value=0
  is_Em8000_settled : MATLAB Function  TreatAsAtomicUnit=on
  OM_traj_points : Outport
  new_command_Out : Outport  Port=2
  OM_Traj_method : Outport  Port=3
  OM_v_max : Outport  Port=4
  Winch_PosRef_Out : Outport  Port=5
  Winch_NewCmd_Out : Outport  Port=6
  FF_Flag : Outport  Port=7
  Winch_Mode_selector_Out : Outport  Port=8
  wires:
  Chart/1(Traj_points_XYZ) -> Operation_Mode_Selector/1(State_Chart_traj_points)
  Operation_Mode_Selector/1(Traj_points_Out) -> OM_traj_points/1  "OM_traj_points"
  Chart/5(Winch_NewCmd) -> Operation_Mode_Selector/6(Winch_NewCmd)
  Constant4/1 -> Chart/2(Switch)  "MS_Switch"
  Chart/8(FF_Flag) -> FF_Flag/1
  Chart/4(v_max) -> Operation_Mode_Selector/4(v_max)
  Chart/6(Winch_PosRef) -> Operation_Mode_Selector/5(Winch_PosRef)
  Chart/3(Traj_method) -> Operation_Mode_Selector/3(Traj_method)
  Chart/2(new_command) -> Operation_Mode_Selector/2(new_command)
  Operation_Mode_Selector/2(new_command_Out) -> new_command_Out/1  "new_command_traj"
  Operation_Mode_Selector/3(Traj_method_Out) -> OM_Traj_method/1  "OM_Traj_method"
  Operation_Mode_Selector/4(v_max_Out) -> OM_v_max/1  "OM_v_max"
  Winch_Local_to_Global/1(Winch_Global_Pos_Z) -> Chart/9(Winch_Pos_world)
  traj_running/1 -> Chart/10(traj_running)
  Operation_Mode_Selector/5(Winch_PosRef_Out) -> Winch_PosRef_Out/1
  bBall_InFrame/1 -> Chart/6(bBall_InFrame)
  Operation_Mode_Selector/6(Winch_NewCmd_Out) -> Winch_NewCmd_Out/1
  Ball_Pos/1 -> Chart/8(Ball_Pos)
  FK_Pos/1 -> Winch_Local_to_Global/1(FK_Pos), Chart/4(FK_Pos)
  Claw_Pos/1 -> Chart/5(Claw_Pos)
  Manual_traj_points/1 -> Operation_Mode_Selector/8(Manual_traj_points)
  Constant/1 -> Chart/1(State_Mode_Selector)
  Chart/7(Winch_Mode_selector) -> Operation_Mode_Selector/7(Winch_Mode_selector)
  Operation_Mode_Selector/7(Winch_Mode_selector_Out) -> Winch_Mode_selector_Out/1
  Winch_length/1 -> Winch_Local_to_Global/2(Winch_Length)
  Em8000_translation/1 -> is_Em8000_settled/1(Em8000_translation)
  is_Em8000_settled/1(Em8000_settled_flag) -> Chart/7(Em8000_settled_flag)  "Em8000_settled_flag"
  enable_65cm_offset_Em8000/1 -> Chart/3(Em8000_comp_offset_flag)

== system sg_IK/Controller/Trajectory planner ==
  OM_traj_points : Inport
  new_command : Inport  Port=2
  OM_Traj_method : Inport  Port=3
  OM_v_max : Inport  Port=4
  Joint_limitFlag : Inport  Port=5
  Clock : Clock
  Demux2 : Demux  Outputs=3
  Memory2 : Memory
  Trajectory_planner : MATLAB Function  TreatAsAtomicUnit=on
  Endeff_traj : Outport
  Endeff_trajvel : Outport  Port=2
  Trajectory_Running_flag : Outport  Port=3
  wires:
  new_command/1 -> Trajectory_planner/5(new_command)
  Trajectory_planner/3(Traj_Running) -> Memory2/1  "Trajectory_Running"
  Clock/1 -> Trajectory_planner/4(t)
  Trajectory_planner/1(p) -> Endeff_traj/1  "Endeff_trajworld"
  Demux2/1 -> Trajectory_planner/1(points_x)
  Demux2/3 -> Trajectory_planner/3(points_z)
  Demux2/2 -> Trajectory_planner/2(points_y)
  OM_Traj_method/1 -> Trajectory_planner/6(traj_method)
  Memory2/1 -> Trajectory_Running_flag/1
  OM_v_max/1 -> Trajectory_planner/7(v_max)
  OM_traj_points/1 -> Demux2/1
  Trajectory_planner/2(p_vel) -> Endeff_trajvel/1  "Endeff_trajvel"
  Joint_limitFlag/1 -> Trajectory_planner/8(Joint_limitFlag)

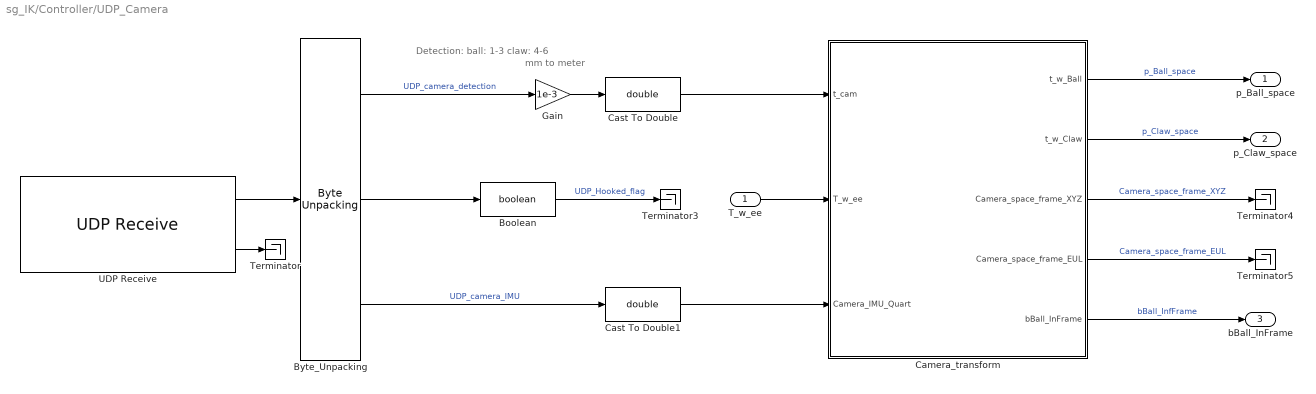
== system sg_IK/Controller/UDP_Camera ==
  note: mm to meter
  note: Detection:
      | ball: 1-3
      | claw: 4-6
  T_w_ee : Inport
  Boolean : DataTypeConversion  OutDataTypeStr=boolean
  Byte_Unpacking : slrealtimeutilitieslib/Byte Unpacking  MaskUnpackedDataTypes={'int16', 'uint8', 'single'}  MaskUnpackedDataSizes={[6], [1], [4]}  MaskAlignment=1
      settings: SourceProductBaseCode=XP
  Camera_transform : MATLAB Function  TreatAsAtomicUnit=on
  Cast To Double : DataTypeConversion  OutDataTypeStr=double
  Cast To Double1 : DataTypeConversion  OutDataTypeStr=double
  Gain : Gain  Gain=1e-3
  Terminator{,3..5} (4 alike) : Terminator
  UDP Receive : slrealtimeiplib/UDP Receive  useHostTargetConn=on  ipAddress=192.168.80.15  localPort=5008  rcvWidth=29  rcvFmAny=on  fmAddress='192.168.80.10'  sampleTime=Ts
      settings: SourceProductBaseCode=XP
  p_Ball_space : Outport
  p_Claw_space : Outport  Port=2
  bBall_InFrame : Outport  Port=3
  wires:
  UDP Receive/2 -> Terminator/1
  UDP Receive/1 -> Byte_Unpacking/1
  Byte_Unpacking/2 -> Boolean/1
  Byte_Unpacking/3 -> Cast To Double1/1  "UDP_camera_IMU"
  Byte_Unpacking/1 -> Gain/1  "UDP_camera_detection"
  Boolean/1 -> Terminator3/1  "UDP_Hooked_flag"
  Gain/1 -> Cast To Double/1
  Camera_transform/1(t_w_Ball) -> p_Ball_space/1  "p_Ball_space"
  Camera_transform/2(t_w_Claw) -> p_Claw_space/1  "p_Claw_space"
  Camera_transform/4(Camera_space_frame_EUL) -> Terminator5/1  "Camera_space_frame_EUL"
  Camera_transform/3(Camera_space_frame_XYZ) -> Terminator4/1  "Camera_space_frame_XYZ"
  Cast To Double/1 -> Camera_transform/1(t_cam)
  Cast To Double1/1 -> Camera_transform/3(Camera_IMU_Quart)
  Camera_transform/5(bBall_InFrame) -> bBall_InFrame/1  "bBall_InfFrame"
  T_w_ee/1 -> Camera_transform/2(T_w_ee)

== system sg_IK/Controller/Winch_Controller ==
  Winch_PosRef : Inport
  Winch_NewCmd : Inport  Port=2
  FF_Flag : Inport  Port=3
  Winch_Mode_selector : Inport  Port=4
  MotionLab_RxUDP_bus : Inport  Port=5
  FK_pos : Inport  Port=6
  Multiport Switch1 : MultiPortSwitch  Inputs=2
  Winch_Camera_Based_HeaveComp : Subsystem
  Winch_StewartFB_Based_HeaveComp : Subsystem
  Winch_Vel_Cmd : Outport
  wires:
  FK_pos/1 -> Winch_Camera_Based_HeaveComp/1(FK_pos), Winch_StewartFB_Based_HeaveComp/1(FK_Pos)
  Winch_PosRef/1 -> Winch_StewartFB_Based_HeaveComp/2(Winch_PosRef), Winch_Camera_Based_HeaveComp/2(Winch_PosRef_camera)
  MotionLab_RxUDP_bus/1 -> Winch_Camera_Based_HeaveComp/3(MotionLab_RxUDP_bus), Winch_StewartFB_Based_HeaveComp/3(MotionLab_RxUDP_bus)
  FF_Flag/1 -> Winch_Camera_Based_HeaveComp/4(FF_Flag), Winch_StewartFB_Based_HeaveComp/4(FF_Flag)
  Winch_Camera_Based_HeaveComp/1(Winch_Vel_Cmd) -> Multiport Switch1/2
  Winch_NewCmd/1 -> Winch_StewartFB_Based_HeaveComp/5(Winch_NewCmd)
  Winch_Mode_selector/1 -> Multiport Switch1/1
  Winch_StewartFB_Based_HeaveComp/1(Winch_Vel_Cmd) -> Multiport Switch1/3
  Multiport Switch1/1 -> Winch_Vel_Cmd/1

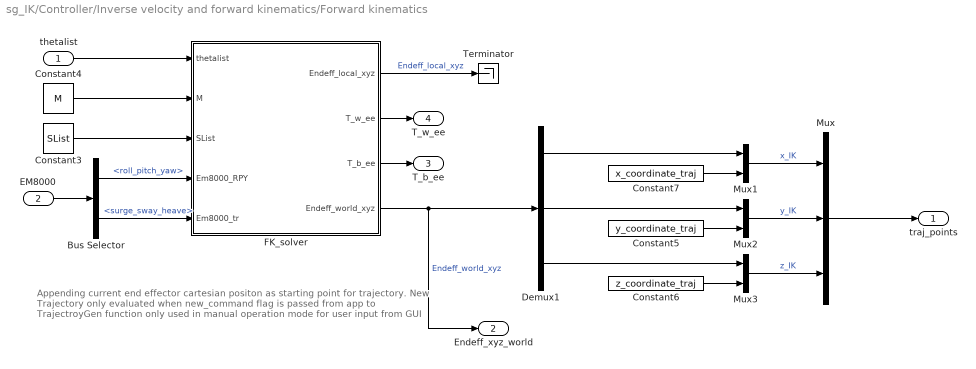
== system sg_IK/Controller/Inverse velocity and forward kinematics/Forward kinematics ==
  note: Appending current end effector cartesian positon
      | as starting point for trajectory. New Trajectory only
      | evaluated when new_command flag is passed from app to TrajectroyGen function
      |
      | only used in manual operation mode for user input from GUI
  thetalist : Inport
  EM8000 : Inport  Port=2
  Bus Selector : BusSelector  OutputSignals=roll_pitch_yaw,surge_sway_heave
  Constant3 : Constant  Value=SList
  Constant4 : Constant  Value=M
  Constant5 : Constant  Value=y_coordinate_traj
  Constant6 : Constant  Value=z_coordinate_traj
  Constant7 : Constant  Value=x_coordinate_traj
  Demux1 : Demux  Outputs=3
  FK_solver : MATLAB Function  TreatAsAtomicUnit=on
  Mux : Mux  Inputs=3
  Mux1 : Mux  Inputs=2
  Mux2 : Mux  Inputs=2
  Mux3 : Mux  Inputs=2
  Terminator : Terminator
  traj_points : Outport
  Endeff_xyz_world : Outport  Port=2
  T_b_ee : Outport  Port=3
  T_w_ee : Outport  Port=4
  wires:
  Demux1/3 -> Mux3/1
  Demux1/1 -> Mux1/1
  Demux1/2 -> Mux2/1
  Constant3/1 -> FK_solver/3(SList)
  Constant4/1 -> FK_solver/2(M)
  FK_solver/4(Endeff_world_xyz) -> Demux1/1, Endeff_xyz_world/1  "Endeff_world_xyz"
  thetalist/1 -> FK_solver/1(thetalist)
  Constant7/1 -> Mux1/2
  Constant5/1 -> Mux2/2
  Constant6/1 -> Mux3/2
  Mux3/1 -> Mux/3  "z_IK"
  Mux2/1 -> Mux/2  "y_IK"
  Mux1/1 -> Mux/1  "x_IK"
  Mux/1 -> traj_points/1
  FK_solver/3(T_b_ee) -> T_b_ee/1
  FK_solver/1(Endeff_local_xyz) -> Terminator/1  "Endeff_local_xyz"
  EM8000/1 -> Bus Selector/1
  Bus Selector/2 -> FK_solver/5(Em8000_tr)  "<surge_sway_heave>"
  Bus Selector/1 -> FK_solver/4(Em8000_RPY)  "<roll_pitch_yaw>"
  FK_solver/2(T_w_ee) -> T_w_ee/1

== system sg_IK/Controller/Inverse velocity and forward kinematics/Theta3 = (Theta3*+90deg) + Theta2 ==
  note: Keep dummy frames always aligned with world axis
  note: q3 = q3* + q2
  MotionLab_RxUDP_bus : Inport
  Bus Selector : BusSelector  OutputSignals=Comau.Theta(1-3)
  Constant : Constant  Value=0
  Constant1 : Constant  Value=0
  Demux : Demux  Outputs=3
  Mux : Mux  Inputs=5
  Sum : Sum  Inputs=|++
  Sum3 : Sum  Inputs=|++
  rad_90degrees : Constant  Value=1.57
  thetalist : Outport
  wires:
  Sum3/1 -> Mux/3
  Sum/1 -> Sum3/1
  Demux/1 -> Mux/1
  Demux/2 -> Mux/2, Sum3/2
  Constant/1 -> Mux/4
  Constant1/1 -> Mux/5
  Mux/1 -> thetalist/1
  rad_90degrees/1 -> Sum/2
  Demux/3 -> Sum/1
  MotionLab_RxUDP_bus/1 -> Bus Selector/1
  Bus Selector/1 -> Demux/1  "<Theta(1-3)>"

== system sg_IK/Controller/Inverse velocity and forward kinematics/ThetaDot3*=ThetaDot3-ThetaDot2 ==
  note: theta_3p = theta_3 - theta_2
  thetaListDot : Inport
  Demux2 : Demux  Outputs=5
  Mux4 : Mux  Inputs=3
  Sum2 : Sum  Inputs=|+-
  Terminator8 : Terminator
  Terminator9 : Terminator
  Out1 : Outport
  wires:
  Demux2/1 -> Mux4/1
  Demux2/3 -> Sum2/1
  Demux2/5 -> Terminator8/1
  Demux2/2 -> Mux4/2, Sum2/2
  Demux2/4 -> Terminator9/1
  Sum2/1 -> Mux4/3
  Mux4/1 -> Out1/1
  thetaListDot/1 -> Demux2/1

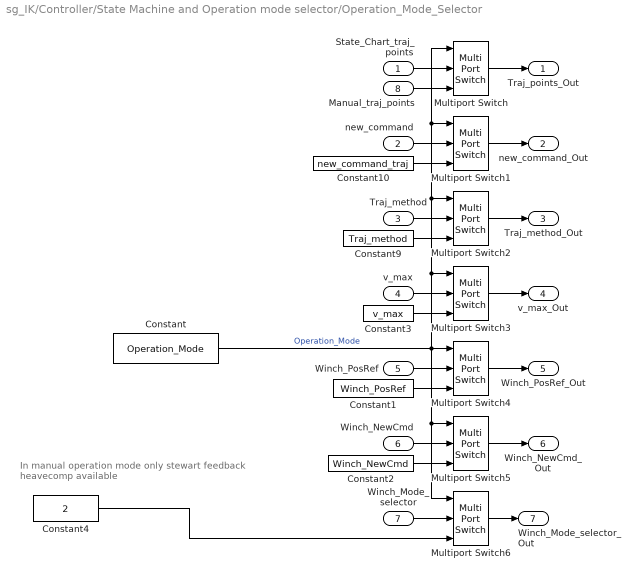
== system sg_IK/Controller/State Machine and Operation mode selector/Operation_Mode_Selector ==
  note: In manual operation mode only stewart
      | feedback heavecomp available
  State_Chart_traj_points : Inport
  new_command : Inport  Port=2
  Traj_method : Inport  Port=3
  v_max : Inport  Port=4
  Winch_PosRef : Inport  Port=5
  Winch_NewCmd : Inport  Port=6
  Winch_Mode_selector : Inport  Port=7
  Manual_traj_points : Inport  Port=8
  Constant : Constant  Value=Operation_Mode
  Constant1 : Constant  Value=Winch_PosRef
  Constant10 : Constant  Value=new_command_traj
  Constant2 : Constant  Value=Winch_NewCmd
  Constant3 : Constant  Value=v_max
  Constant4 : Constant  Value=2
  Constant9 : Constant  Value=Traj_method
  Multiport Switch{,1..6} (7 alike) : MultiPortSwitch  DataPortOrder=Specify indices  Inputs=2  DataPortIndices={1,2}
  Traj_points_Out : Outport
  new_command_Out : Outport  Port=2
  Traj_method_Out : Outport  Port=3
  v_max_Out : Outport  Port=4
  Winch_PosRef_Out : Outport  Port=5
  Winch_NewCmd_Out : Outport  Port=6
  Winch_Mode_selector_Out : Outport  Port=7
  wires:
  Constant3/1 -> Multiport Switch3/3
  Constant/1 -> Multiport Switch/1, Multiport Switch1/1, Multiport Switch2/1, Multiport Switch3/1, Multiport Switch5/1, Multiport Switch6/1, Multiport Switch4/1  "Operation_Mode"
  Multiport Switch3/1 -> v_max_Out/1
  Multiport Switch1/1 -> new_command_Out/1
  Manual_traj_points/1 -> Multiport Switch/3
  Constant10/1 -> Multiport Switch1/3
  Constant9/1 -> Multiport Switch2/3
  Multiport Switch2/1 -> Traj_method_Out/1
  Multiport Switch/1 -> Traj_points_Out/1
  Constant1/1 -> Multiport Switch4/3
  Multiport Switch4/1 -> Winch_PosRef_Out/1
  State_Chart_traj_points/1 -> Multiport Switch/2
  new_command/1 -> Multiport Switch1/2
  Traj_method/1 -> Multiport Switch2/2
  v_max/1 -> Multiport Switch3/2
  Winch_PosRef/1 -> Multiport Switch4/2
  Multiport Switch5/1 -> Winch_NewCmd_Out/1
  Constant2/1 -> Multiport Switch5/3
  Winch_NewCmd/1 -> Multiport Switch5/2
  Multiport Switch6/1 -> Winch_Mode_selector_Out/1
  Constant4/1 -> Multiport Switch6/3
  Winch_Mode_selector/1 -> Multiport Switch6/2

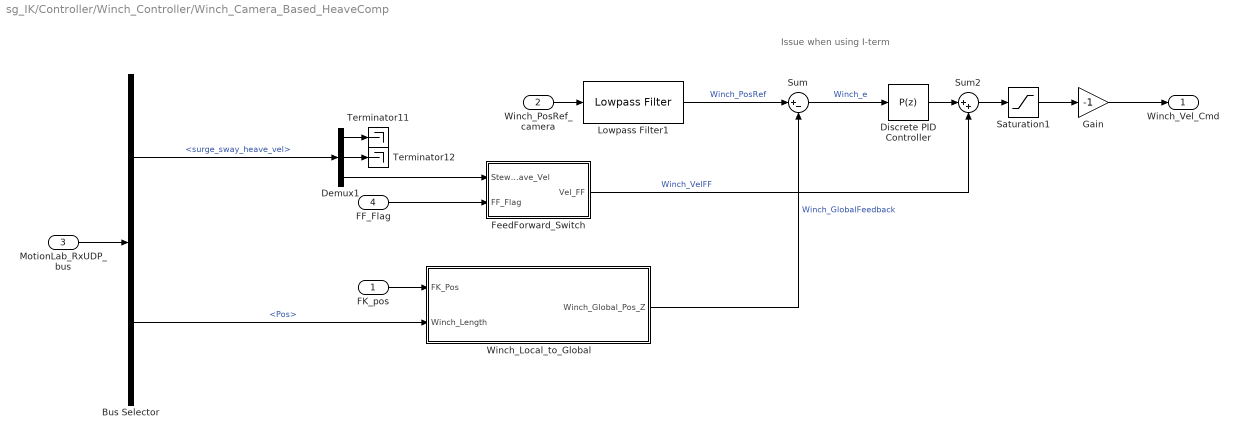
== system sg_IK/Controller/Winch_Controller/Winch_Camera_Based_HeaveComp ==
  note: Issue when using I-term
  FK_pos : Inport
  Winch_PosRef_camera : Inport  Port=2
  MotionLab_RxUDP_bus : Inport  Port=3
  FF_Flag : Inport  Port=4
  Bus Selector : BusSelector  OutputSignals=Em1500.surge_sway_heave_vel,Comau_winch.Pos
  Demux1 : Demux  Outputs=3
  Discrete PID Controller : slpidlib/PID Controller  Controller=P  Form=Parallel  TimeDomain=Discrete-time  UseExternalTs=off  SampleTime=Ts  IntegratorMethod=Forward Euler  FilterMethod=Forward Euler  ControllerParametersSource=internal  P=2  I=0.09  D=0  UseFilter=on  N=100  TunerSelectOption=Transfer Function Based (PID Tuner App)  InitialConditionSource=internal  InitialConditionForIntegrator=0  InitialConditionForFilter=0  DifferentiatorICPrevScaledInput=0  ExternalReset=none  TrackingMode=off  Kt=1  LimitOutput=off  SatLimitsSource=internal  UpperSaturationLimit=inf  LowerSaturationLimit=-inf  LinearizeAsGain=off  AntiWindupMode=none  Kb=1  POutMin=[]  POutMax=[]  IOutMin=[]  IOutMax=[]  DOutMin=[]  DOutMax=[]  NOutMin=[]  NOutMax=[]  SumOutMin=[]  SumOutMax=[]  SaturationOutMin=[]  SaturationOutMax=[]  PParamMin=[]  PParamMax=[]  IParamMin=[]  IParamMax=[]  DParamMin=[]  DParamMax=[]  NParamMin=[]  NParamMax=[]  KbParamMin=[]  KbParamMax=[]  KtParamMin=[]  KtParamMax=[]  KbOutMin=[]  KbOutMax=[]  KtOutMin=[]  KtOutMax=[]  IntegratorOutMin=[]  IntegratorOutMax=[]  FilterOutMin=[]  FilterOutMax=[]  SumI1OutMin=[]  SumI1OutMax=[]  SumI2OutMin=[]  SumI2OutMax=[]  SumI3OutMin=[]  SumI3OutMax=[]  SumI4OutMin=[]  SumI4OutMax=[]  SumDOutMin=[]  SumDOutMax=[]  DifferentiatorOutMin=[]  DifferentiatorOutMax=[]  FilterDiffOutCoefMin=[]  FilterDiffOutCoefMax=[]  ReciprocalOutMin=[]  ReciprocalOutMax=[]  SumDenOutMin=[]  SumDenOutMax=[]  SumNumOutMin=[]  SumNumOutMax=[]  DivideOutMin=[]  DivideOutMax=[]  UdiffTsProdOutMin=[]  UdiffTsProdOutMax=[]  NTsProdOutMin=[]  NTsProdOutMax=[]  UintegralTsProdOutMin=[]  UintegralTsProdOutMax=[]  UngainTsProdOutMin=[]  UngainTsProdOutMax=[]  FilterDenConstantOutDataTypeStr=Inherit: Inherit via back propagation  FilterDenConstantOutMin=[]  FilterDenConstantOutMax=[]  PCopyOutDataTypeStr=Inherit: Inherit via back propagation  PCopyOutMin=[]  PCopyOutMax=[]  NCopyOutDataTypeStr=Inherit: Inherit via back propagation  NCopyOutMin=[]  NCopyOutMax=[]  IntegratorContinuousStateAttributes=''  IntegratorStateMustResolveToSignalObject=off  IntegratorRTWStateStorageClass=Auto  FilterContinuousStateAttributes=''  FilterStateMustResolveToSignalObject=off  FilterRTWStateStorageClass=Auto  ParallelPVariant=InternalParameters  IdealPVariant=Disabled  IVariant=Disabled  DVariant=Disabled  IntegratorVariant=Disabled  SatVariant=Disabled  AWVariant=Disabled  PCopyVariant=Disabled  TRVariant=Disabled  FdbkBlocksVariant=Forward  IdealPFdbkVariant=Disabled  SatFdbkVariant=Disabled  DerivativeFilterVariant=Disabled  NVariant=Disabled  NCopyVariant=Disabled_SignalSpec  FilterICVariant=Disabled  IntegratorICVariant=Disabled  ExternalResetVariant=Disabled  TRSumVariant=Passthrough  SumFdbkVariant=Disabled  SumVariant=Passthrough_P  TsampFilterVariant=InternalTs  TsampNgainVariant=Passthrough  TsampIntegralVariant=Disabled_SignalSpec  ExternalSaturationOutDataTypeStr=Inherit: Same as second input
  FeedForward_Switch : MATLAB Function  TreatAsAtomicUnit=on
  Gain : Gain  Gain=-1
  Lowpass Filter1 : dspfdesign/Lowpass Filter  FilterType=FIR  DesignForMinimumOrder=on  FilterOrder=50  PassbandFrequency=0.5  StopbandFrequency=3  PassbandRipple=0.5  StopbandAttenuation=40  InheritSampleRate=on  SampleRate=44100  SimulateUsing=Interpreted execution  roundingMode=Floor  coeffsDataTypeStr=fixdt(1,16)
  Saturation1 : Saturate  UpperLimit=0.2  LowerLimit=-0.2
  Sum : Sum  Inputs=|+-
  Sum2 : Sum  Inputs=|++
  Terminator11 : Terminator
  Terminator12 : Terminator
  Winch_Local_to_Global : MATLAB Function  TreatAsAtomicUnit=on
  Winch_Vel_Cmd : Outport
  wires:
  Lowpass Filter1/1 -> Sum/1  "Winch_PosRef"
  Sum/1 -> Discrete PID Controller/1  "Winch_e"
  Saturation1/1 -> Gain/1
  Discrete PID Controller/1 -> Sum2/1
  Bus Selector/2 -> Winch_Local_to_Global/2(Winch_Length)  "<Pos>"
  Demux1/2 -> Terminator12/1
  Sum2/1 -> Saturation1/1
  Bus Selector/1 -> Demux1/1  "<surge_sway_heave_vel>"
  Gain/1 -> Winch_Vel_Cmd/1
  Winch_Local_to_Global/1(Winch_Global_Pos_Z) -> Sum/2  "Winch_GlobalFeedback"
  MotionLab_RxUDP_bus/1 -> Bus Selector/1
  Demux1/1 -> Terminator11/1
  FF_Flag/1 -> FeedForward_Switch/2(FF_Flag)
  FK_pos/1 -> Winch_Local_to_Global/1(FK_Pos)
  Demux1/3 -> FeedForward_Switch/1(Stewart_Heave_Vel)
  Winch_PosRef_camera/1 -> Lowpass Filter1/1
  FeedForward_Switch/1(Vel_FF) -> Sum2/2  "Winch_VelFF"
